simulink model "ECGdenoising_systemgenerator"  (R2018a)
settings: Solver=VariableStepAuto  StartTime=0.0  StopTime=10800  RelTol=1e-3
libraries: xbsIndex_r4 x811, dspsrcs4 x1
(part 1 of 3)
settings Model: Creator=NIKHIL  LastModifiedBy=NIKHIL

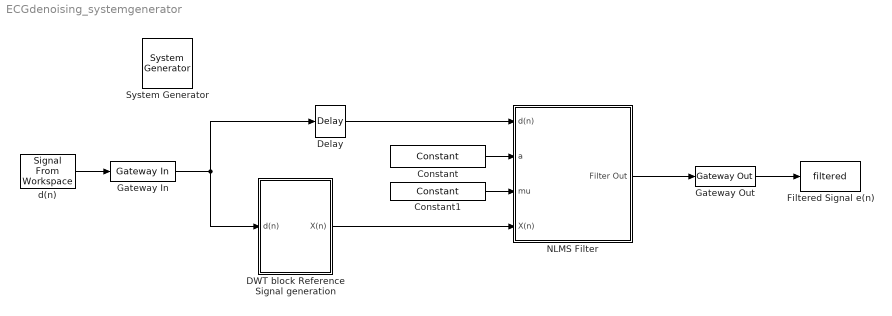
== system ECGdenoising_systemgenerator ==
  " System Generator" : xbsIndex_r4/ System Generator  Tag=genX  xilinxfamily=virtex7  part=xc7vx485t  speed=-2  package=ffg1761  synthesis_tool=Vivado  clock_wrapper=Clock Enables  directory=C:/Users/NIKHIL/Desktop/HDLCODE  proj_type=Vivado  Synth_file=Vivado Synthesis Defaults  Impl_file=Vivado Implementation Defaults  testbench=on  simulink_period=1  sysclk_period=10  dcm_input_clock_period=10  incr_netlist=off  trim_vbits=Everywhere in SubSystem  dbl_ovrd=According to Block Masks  core_generation=According to Block Masks  run_coregen=off  deprecated_control=off  eval_field=0  block_type=sysgen
  Constant : xbsIndex_r4/Constant  const=0.091  gui_display_data_type=Fixed-point  arith_type=Signed (2's comp)  n_bits=16  bin_pt=14  preci_type=Single  exp_width=8  frac_width=24  explicit_period=on  period=1  equ=P=C  opselect=C  inp2=PCIN>>17  opr=+  inp1=P  carry=CIN  dbl_ovrd=off  block_type=constant
  Constant1 : xbsIndex_r4/Constant  const=0.01  gui_display_data_type=Fixed-point  arith_type=Signed (2's comp)  n_bits=16  bin_pt=14  preci_type=Single  exp_width=8  frac_width=24  explicit_period=on  period=1  equ=P=C  opselect=C  inp2=PCIN>>17  opr=+  inp1=P  carry=CIN  dbl_ovrd=off  block_type=constant
  DWT block Reference Signal generation : Subsystem
  Delay : xbsIndex_r4/Delay  rst=off  infoeditControl=Selection of Reset will increase slice count due to use of real FFs and instead of SRLs  en=off  latency=889  reg_retiming=off  dbl_ovrd=off  block_type=delay
  Filtered Signal e(n) : ToWorkspace  VariableName=filtered  SampleTime=1
      settings: Save2DSignal=2-D array (concatenate along first dimension)
  Gateway In : xbsIndex_r4/Gateway In  gui_display_data_type=Fixed-point  arith_type="Signed  (2's comp)"  n_bits=16  bin_pt=14  preci_type=Single  exp_width=8  frac_width=24  rows=1  columns=1  quantization="Round  (unbiased: +/- Inf)"  overflow=Saturate  period=1  UseAsADC=off  ADCChannel='1'  interface=None  automatic_assignment=on  address_offset=hex2dec('00')  intf_name=''  intf_description=''  default_value=0  timing_constraint=None  locs_specified=off  LOCs={}  io_standard={}  inherit_from_input=off  hdl_port=on  dbl_ovrd=off  block_type=gatewayin
  Gateway Out : xbsIndex_r4/Gateway Out  inherit_from_input=off  hdl_port=on  rows=1  columns=1  UseAsDAC=off  DACChannel='1'  interface=None  automatic_assignment=on  address_offset=hex2dec('00')  intf_name=''  intf_description=''  timing_constraint=None  locs_specified=off  LOCs={}  io_standard={}  block_type=gatewayout
  NLMS Filter : Subsystem
  "d(n) " : dspsrcs4/Signal From Workspace  X=din  Ts=1  nsamps=1  OutputAfterFinalValue=Setting to zero  ignoreOrWarnInputAndFrameLengths=off  OutputFrames=off
  wires:
  Constant1/1 -> NLMS Filter/3(mu)
  NLMS Filter/1(Filter Out) -> Gateway Out/1
  "d(n) "/1 -> Gateway In/1
  Constant/1 -> NLMS Filter/2(a)
  DWT block Reference Signal generation/1(X(n)) -> NLMS Filter/4(X(n))
  Gateway Out/1 -> Filtered Signal e(n)/1
  Gateway In/1 -> DWT block Reference Signal generation/1("d(n) "), Delay/1
  Delay/1 -> NLMS Filter/1(d(n))

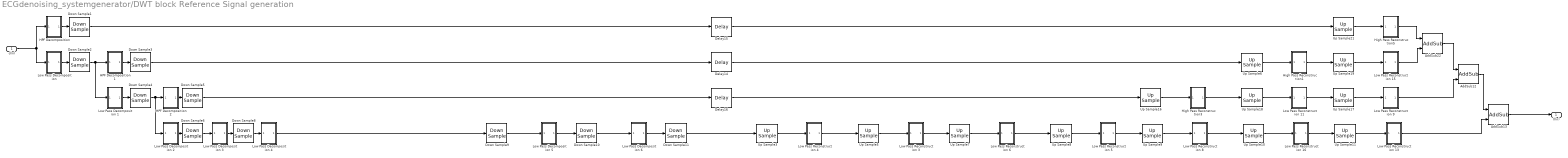
== system ECGdenoising_systemgenerator/DWT block Reference Signal generation ==
  "d(n) " : Inport  SampleTime=1
  AddSub12 : xbsIndex_r4/AddSub  mode=Addition  use_carryin=off  use_carryout=off  en=off  latency=0  precision=User Defined  arith_type="Signed  (2's comp)"  n_bits=16  bin_pt=14  quantization=Truncate  overflow=Saturate  use_behavioral_HDL=off  hw_selection=Fabric  pipelined=off  dbl_ovrd=off  block_type=addsub
  AddSub13 : xbsIndex_r4/AddSub  mode=Addition  use_carryin=off  use_carryout=off  en=off  latency=0  precision=User Defined  arith_type="Signed  (2's comp)"  n_bits=16  bin_pt=14  quantization=Truncate  overflow=Saturate  use_behavioral_HDL=off  hw_selection=Fabric  pipelined=off  dbl_ovrd=off  block_type=addsub
  AddSub22 : xbsIndex_r4/AddSub  mode=Addition  use_carryin=off  use_carryout=off  en=off  latency=0  precision=User Defined  arith_type="Signed  (2's comp)"  n_bits=16  bin_pt=14  quantization=Truncate  overflow=Saturate  use_behavioral_HDL=off  hw_selection=Fabric  pipelined=off  dbl_ovrd=off  block_type=addsub
  Delay14 : xbsIndex_r4/Delay  rst=off  infoeditControl=Selection of Reset will increase slice count due to use of real FFs and instead of SRLs  en=off  latency=217  reg_retiming=off  dbl_ovrd=off  block_type=delay
  Delay15 : xbsIndex_r4/Delay  rst=off  infoeditControl=Selection of Reset will increase slice count due to use of real FFs and instead of SRLs  en=off  latency=441  reg_retiming=off  dbl_ovrd=off  block_type=delay
  Delay16 : xbsIndex_r4/Delay  rst=off  infoeditControl=Selection of Reset will increase slice count due to use of real FFs and instead of SRLs  en=off  latency=105  reg_retiming=off  dbl_ovrd=off  block_type=delay
  Down Sample{1..6,8..11} (10 alike) : xbsIndex_r4/Down Sample  sample_ratio=2  sample_phase=First Value of Frame  en=off  rst=off  latency=0  dbl_ovrd=off  block_type=dsamp
  "HPF Decomposition " : Subsystem
  HPF Decomposition 1 : Subsystem
  HPF Decomposition 2 : Subsystem
  High Pass Reconstruction1 : Subsystem
  High Pass Reconstruction3 : Subsystem
  High Pass Reconstruction5 : Subsystem
  "Low Pass Decomposition " : Subsystem
  Low Pass Decomposition 1 : Subsystem
  Low Pass Decomposition 2 : Subsystem
  Low Pass Decomposition 3 : Subsystem
  Low Pass Decomposition 4 : Subsystem
  Low Pass Decomposition 5 : Subsystem
  Low Pass Decomposition 6 : Subsystem
  Low Pass Reconstruction 11 : Subsystem
  Low Pass Reconstruction 13 : Subsystem
  Low Pass Reconstruction 15 : Subsystem
  Low Pass Reconstruction 16 : Subsystem
  Low Pass Reconstruction 3 : Subsystem
  Low Pass Reconstruction 4 : Subsystem
  Low Pass Reconstruction 5 : Subsystem
  Low Pass Reconstruction 6 : Subsystem
  Low Pass Reconstruction 8 : Subsystem
  Low Pass Reconstruction 9 : Subsystem
  Up Sample{3,5..11,16..19,21} (13 alike) : xbsIndex_r4/Up Sample  sample_ratio=2  copy_samples=off  en=off  latency=0  dbl_ovrd=off  block_type=usamp
  X(n) : Outport  SampleTime=1
  wires:
  Down Sample3/1 -> Delay14/1
  Up Sample10/1 -> Low Pass Reconstruction 16/1(In3)
  AddSub22/1 -> AddSub12/1
  Down Sample5/1 -> Delay16/1
  Low Pass Reconstruction 15/1(Out3) -> AddSub22/2
  Up Sample6/1 -> High Pass Reconstruction1/1(In4)
  Low Pass Reconstruction 13/1(Out3) -> AddSub13/2
  Low Pass Reconstruction 5/1(Out3) -> Up Sample9/1
  Low Pass Reconstruction 9/1(Out3) -> AddSub12/2
  Up Sample11/1 -> Low Pass Reconstruction 13/1(In3)
  High Pass Reconstruction5/1(Out4) -> AddSub22/1
  Low Pass Reconstruction 8/1(Out3) -> Up Sample10/1
  High Pass Reconstruction1/1(Out4) -> Up Sample19/1
  AddSub13/1 -> X(n)/1
  Low Pass Reconstruction 3/1(Out3) -> Up Sample7/1
  Up Sample16/1 -> High Pass Reconstruction3/1(In4)
  Down Sample11/1 -> Up Sample3/1
  Up Sample8/1 -> Low Pass Reconstruction 5/1(In3)
  Up Sample18/1 -> Low Pass Reconstruction 11/1(In3)
  Delay15/1 -> Up Sample21/1
  Up Sample7/1 -> Low Pass Reconstruction 6/1(In3)
  Low Pass Reconstruction 6/1(Out3) -> Up Sample8/1
  Up Sample5/1 -> Low Pass Reconstruction 3/1(In3)
  Up Sample19/1 -> Low Pass Reconstruction 15/1(In3)
  Down Sample4/1 -> Low Pass Decomposition 2/1(In1), HPF Decomposition 2/1(In2)
  High Pass Reconstruction3/1(Out4) -> Up Sample18/1
  Up Sample3/1 -> Low Pass Reconstruction 4/1(In3)
  "HPF Decomposition "/1(Out2) -> Down Sample1/1
  Down Sample9/1 -> Low Pass Decomposition 5/1(In1)
  Low Pass Decomposition 4/1(Out1) -> Down Sample9/1
  Low Pass Reconstruction 16/1(Out3) -> Up Sample11/1
  Low Pass Decomposition 1/1(Out1) -> Down Sample4/1
  Down Sample8/1 -> Low Pass Decomposition 4/1(In1)
  Low Pass Decomposition 2/1(Out1) -> Down Sample6/1
  Low Pass Decomposition 3/1(Out1) -> Down Sample8/1
  Low Pass Decomposition 6/1(Out1) -> Down Sample11/1
  Up Sample21/1 -> High Pass Reconstruction5/1(In4)
  Low Pass Reconstruction 11/1(Out3) -> Up Sample17/1
  Low Pass Decomposition 5/1(Out1) -> Down Sample10/1
  Up Sample9/1 -> Low Pass Reconstruction 8/1(In3)
  Delay16/1 -> Up Sample16/1
  Down Sample2/1 -> Low Pass Decomposition 1/1(In1), HPF Decomposition 1/1(In2)
  HPF Decomposition 2/1(Out2) -> Down Sample5/1
  Delay14/1 -> Up Sample6/1
  AddSub12/1 -> AddSub13/1
  Up Sample17/1 -> Low Pass Reconstruction 9/1(In3)
  Down Sample10/1 -> Low Pass Decomposition 6/1(In1)
  Low Pass Reconstruction 4/1(Out3) -> Up Sample5/1
  "Low Pass Decomposition "/1(Out1) -> Down Sample2/1
  Down Sample1/1 -> Delay15/1
  "d(n) "/1 -> "HPF Decomposition "/1(In2), "Low Pass Decomposition "/1(In1)
  Down Sample6/1 -> Low Pass Decomposition 3/1(In1)
  HPF Decomposition 1/1(Out2) -> Down Sample3/1

== system ECGdenoising_systemgenerator/NLMS Filter ==
  note: e(n)
  d(n) : Inport  SampleTime=1
  a : Inport  Port=2  SampleTime=1
  mu : Inport  Port=3  SampleTime=1
  X(n) : Inport  Port=4  SampleTime=1
  12 tap FIR Filter : Subsystem
  AddSub12 : xbsIndex_r4/AddSub  mode=Subtraction  use_carryin=off  use_carryout=off  en=off  latency=0  precision=User Defined  arith_type="Signed  (2's comp)"  n_bits=16  bin_pt=14  quantization=Truncate  overflow=Saturate  use_behavioral_HDL=off  hw_selection=Fabric  pipelined=off  dbl_ovrd=off  block_type=addsub
  NLMS Algorithm : Subsystem
  Filter Out : Outport  SampleTime=1
  wires:
  NLMS Algorithm/4(coef4) -> 12 tap FIR Filter/5(Coeff4)
  NLMS Algorithm/9(coef9) -> 12 tap FIR Filter/10(Coeff9)
  mu/1 -> NLMS Algorithm/3(mu)
  AddSub12/1 -> Filter Out/1, NLMS Algorithm/1(e(n))
  12 tap FIR Filter/1(Y(n)) -> AddSub12/2
  X(n)/1 -> 12 tap FIR Filter/1("X(n) "), NLMS Algorithm/4(X(n))
  NLMS Algorithm/10(coef10) -> 12 tap FIR Filter/11(Coeff10)
  NLMS Algorithm/2(coef2) -> 12 tap FIR Filter/3(Coeff2)
  NLMS Algorithm/8(coef8) -> 12 tap FIR Filter/9(Coeff8)
  NLMS Algorithm/6(coef6) -> 12 tap FIR Filter/7(Coeff6)
  NLMS Algorithm/11(coef11) -> 12 tap FIR Filter/12(Coeff11)
  NLMS Algorithm/5(coef5) -> 12 tap FIR Filter/6(Coeff5)
  NLMS Algorithm/7(coef7) -> 12 tap FIR Filter/8(Coeff7)
  NLMS Algorithm/1(coef1) -> 12 tap FIR Filter/2(Coeff1)
  d(n)/1 -> AddSub12/1
  NLMS Algorithm/12(coef12) -> 12 tap FIR Filter/13(Coeff12)
  NLMS Algorithm/3(coef3) -> 12 tap FIR Filter/4(Coeff3)
  a/1 -> NLMS Algorithm/2(a)

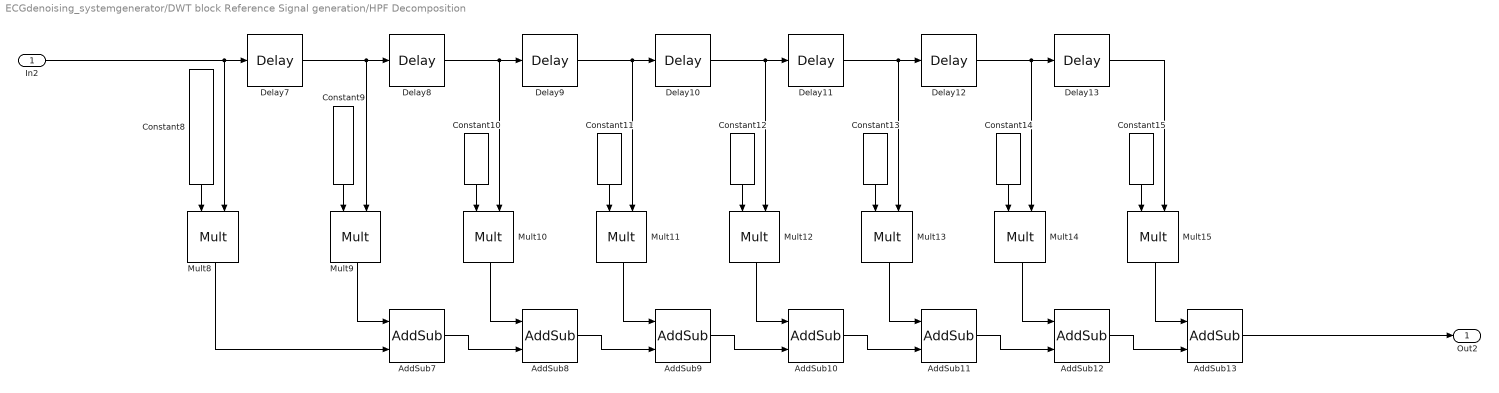
== system ECGdenoising_systemgenerator/DWT block Reference Signal generation/HPF Decomposition  ==
  In2 : Inport
  AddSub{7..13} (7 alike) : xbsIndex_r4/AddSub  mode=Addition  use_carryin=off  use_carryout=off  en=off  latency=0  precision=User Defined  arith_type="Signed  (2's comp)"  n_bits=16  bin_pt=14  quantization=Truncate  overflow=Saturate  use_behavioral_HDL=off  hw_selection=Fabric  pipelined=off  dbl_ovrd=off  block_type=addsub
  Constant10 : xbsIndex_r4/Constant  const=-0.6308807679  gui_display_data_type=Fixed-point  arith_type=Signed (2's comp)  n_bits=16  bin_pt=14  preci_type=Single  exp_width=8  frac_width=24  explicit_period=on  period=1  equ=P=C  opselect=C  inp2=PCIN>>17  opr=+  inp1=P  carry=CIN  dbl_ovrd=off  block_type=constant
  Constant11 : xbsIndex_r4/Constant  const=-0.0279837694  gui_display_data_type=Fixed-point  arith_type=Signed (2's comp)  n_bits=16  bin_pt=14  preci_type=Single  exp_width=8  frac_width=24  explicit_period=on  period=1  equ=P=C  opselect=C  inp2=PCIN>>17  opr=+  inp1=P  carry=CIN  dbl_ovrd=off  block_type=constant
  Constant12 : xbsIndex_r4/Constant  const=0.1870348117  gui_display_data_type=Fixed-point  arith_type=Signed (2's comp)  n_bits=16  bin_pt=14  preci_type=Single  exp_width=8  frac_width=24  explicit_period=on  period=1  equ=P=C  opselect=C  inp2=PCIN>>17  opr=+  inp1=P  carry=CIN  dbl_ovrd=off  block_type=constant
  Constant13 : xbsIndex_r4/Constant  const=0.0308413818  gui_display_data_type=Fixed-point  arith_type=Signed (2's comp)  n_bits=16  bin_pt=14  preci_type=Single  exp_width=8  frac_width=24  explicit_period=on  period=1  equ=P=C  opselect=C  inp2=PCIN>>17  opr=+  inp1=P  carry=CIN  dbl_ovrd=off  block_type=constant
  Constant14 : xbsIndex_r4/Constant  const=-0.0328830117  gui_display_data_type=Fixed-point  arith_type=Signed (2's comp)  n_bits=16  bin_pt=14  preci_type=Single  exp_width=8  frac_width=24  explicit_period=on  period=1  equ=P=C  opselect=C  inp2=PCIN>>17  opr=+  inp1=P  carry=CIN  dbl_ovrd=off  block_type=constant
  Constant15 : xbsIndex_r4/Constant  const=-0.0105974018  gui_display_data_type=Fixed-point  arith_type=Signed (2's comp)  n_bits=16  bin_pt=14  preci_type=Single  exp_width=8  frac_width=24  explicit_period=on  period=1  equ=P=C  opselect=C  inp2=PCIN>>17  opr=+  inp1=P  carry=CIN  dbl_ovrd=off  block_type=constant
  Constant8 : xbsIndex_r4/Constant  const=-0.2303778133  gui_display_data_type=Fixed-point  arith_type=Signed (2's comp)  n_bits=16  bin_pt=14  preci_type=Single  exp_width=8  frac_width=24  explicit_period=on  period=1  equ=P=C  opselect=C  inp2=PCIN>>17  opr=+  inp1=P  carry=CIN  dbl_ovrd=off  block_type=constant
  Constant9 : xbsIndex_r4/Constant  const=0.7148465706  gui_display_data_type=Fixed-point  arith_type=Signed (2's comp)  n_bits=16  bin_pt=14  preci_type=Single  exp_width=8  frac_width=24  explicit_period=on  period=1  equ=P=C  opselect=C  inp2=PCIN>>17  opr=+  inp1=P  carry=CIN  dbl_ovrd=off  block_type=constant
  Delay{7..13} (7 alike) : xbsIndex_r4/Delay  rst=off  infoeditControl=Selection of Reset will increase slice count due to use of real FFs and instead of SRLs  en=off  latency=1  reg_retiming=off  dbl_ovrd=off  block_type=delay
      Delay10 settings: infoedit=Hardware notes: A delay line is a chain, each link of which is an SRL16 or SRL32 followed by a flip-flop.
      Delay11 settings: infoedit=Hardware notes: A delay line is a chain, each link of which is an SRL16 or SRL32 followed by a flip-flop.
      Delay12 settings: infoedit=Hardware notes: A delay line is a chain, each link of which is an SRL16 or SRL32 followed by a flip-flop.
      Delay13 settings: infoedit=Hardware notes: A delay line is a chain, each link of which is an SRL16 or SRL32 followed by a flip-flop.
      Delay7 settings: infoedit=Hardware notes: A delay line is a chain, each link of which is an SRL16 or SRL32 followed by a flip-flop.
      Delay8 settings: infoedit=Hardware notes: A delay line is a chain, each link of which is an SRL16 or SRL32 followed by a flip-flop.
  Mult{8..15} (8 alike) : xbsIndex_r4/Mult  precision=User Defined  arith_type="Signed  (2's comp)"  n_bits=32  bin_pt=28  quantization=Truncate  overflow=Saturate  en=off  latency=0  use_behavioral_HDL=off  opt=Speed  use_embedded=on  optimum_pipeline=off  pipeline=on  dbl_ovrd=off  use_rpm=on  placement_style=Triangular  block_type=mult
  Out2 : Outport
  wires:
  Constant8/1 -> Mult8/1
  Constant9/1 -> Mult9/1
  Constant10/1 -> Mult10/1
  Mult10/1 -> AddSub8/1
  AddSub7/1 -> AddSub8/2
  Delay9/1 -> Mult11/2, Delay10/1
  Constant11/1 -> Mult11/1
  Mult11/1 -> AddSub9/1
  AddSub8/1 -> AddSub9/2
  Mult8/1 -> AddSub7/2
  Delay10/1 -> Mult12/2, Delay11/1
  Delay7/1 -> Mult9/2, Delay8/1
  Mult9/1 -> AddSub7/1
  In2/1 -> Mult8/2, Delay7/1
  Delay8/1 -> Mult10/2, Delay9/1
  Constant13/1 -> Mult13/1
  Delay13/1 -> Mult15/2
  Constant15/1 -> Mult15/1
  Mult15/1 -> AddSub13/1
  Mult13/1 -> AddSub11/1
  AddSub9/1 -> AddSub10/2
  Mult14/1 -> AddSub12/1
  AddSub11/1 -> AddSub12/2
  Mult12/1 -> AddSub10/1
  Delay11/1 -> Mult13/2, Delay12/1
  AddSub10/1 -> AddSub11/2
  Constant14/1 -> Mult14/1
  AddSub12/1 -> AddSub13/2
  Constant12/1 -> Mult12/1
  Delay12/1 -> Mult14/2, Delay13/1
  AddSub13/1 -> Out2/1

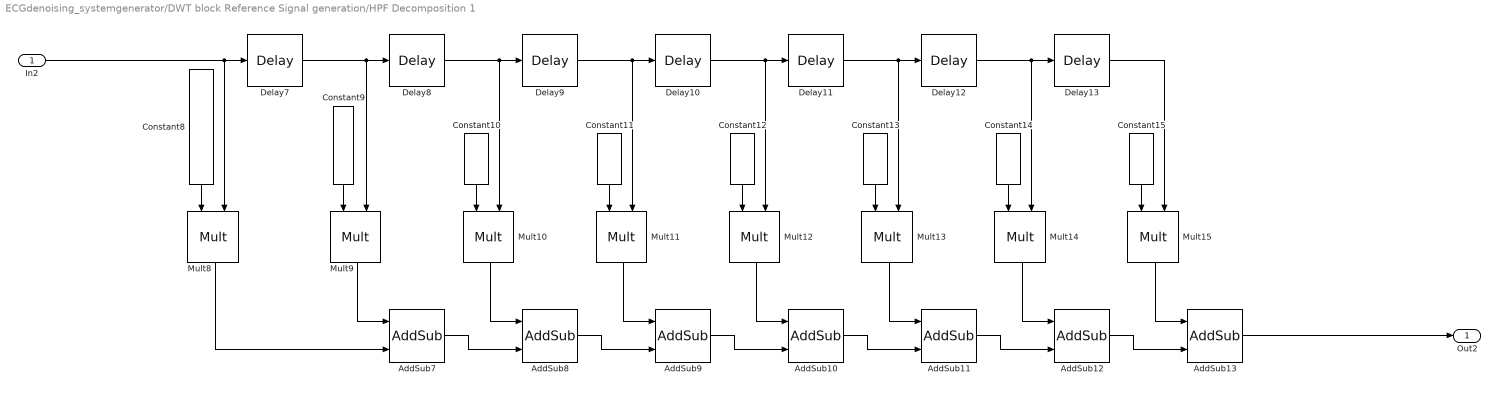
== system ECGdenoising_systemgenerator/DWT block Reference Signal generation/HPF Decomposition 1 ==
  In2 : Inport
  AddSub{7..13} (7 alike) : xbsIndex_r4/AddSub  mode=Addition  use_carryin=off  use_carryout=off  en=off  latency=0  precision=User Defined  arith_type="Signed  (2's comp)"  n_bits=16  bin_pt=14  quantization=Truncate  overflow=Saturate  use_behavioral_HDL=off  hw_selection=Fabric  pipelined=off  dbl_ovrd=off  block_type=addsub
  Constant10 : xbsIndex_r4/Constant  const=-0.6308807679  gui_display_data_type=Fixed-point  arith_type=Signed (2's comp)  n_bits=16  bin_pt=14  preci_type=Single  exp_width=8  frac_width=24  explicit_period=on  period=2  equ=P=C  opselect=C  inp2=PCIN>>17  opr=+  inp1=P  carry=CIN  dbl_ovrd=off  block_type=constant
  Constant11 : xbsIndex_r4/Constant  const=-0.0279837694  gui_display_data_type=Fixed-point  arith_type=Signed (2's comp)  n_bits=16  bin_pt=14  preci_type=Single  exp_width=8  frac_width=24  explicit_period=on  period=2  equ=P=C  opselect=C  inp2=PCIN>>17  opr=+  inp1=P  carry=CIN  dbl_ovrd=off  block_type=constant
  Constant12 : xbsIndex_r4/Constant  const=0.1870348117  gui_display_data_type=Fixed-point  arith_type=Signed (2's comp)  n_bits=16  bin_pt=14  preci_type=Single  exp_width=8  frac_width=24  explicit_period=on  period=2  equ=P=C  opselect=C  inp2=PCIN>>17  opr=+  inp1=P  carry=CIN  dbl_ovrd=off  block_type=constant
  Constant13 : xbsIndex_r4/Constant  const=0.0308413818  gui_display_data_type=Fixed-point  arith_type=Signed (2's comp)  n_bits=16  bin_pt=14  preci_type=Single  exp_width=8  frac_width=24  explicit_period=on  period=2  equ=P=C  opselect=C  inp2=PCIN>>17  opr=+  inp1=P  carry=CIN  dbl_ovrd=off  block_type=constant
  Constant14 : xbsIndex_r4/Constant  const=-0.0328830117  gui_display_data_type=Fixed-point  arith_type=Signed (2's comp)  n_bits=16  bin_pt=14  preci_type=Single  exp_width=8  frac_width=24  explicit_period=on  period=2  equ=P=C  opselect=C  inp2=PCIN>>17  opr=+  inp1=P  carry=CIN  dbl_ovrd=off  block_type=constant
  Constant15 : xbsIndex_r4/Constant  const=-0.0105974018  gui_display_data_type=Fixed-point  arith_type=Signed (2's comp)  n_bits=16  bin_pt=14  preci_type=Single  exp_width=8  frac_width=24  explicit_period=on  period=2  equ=P=C  opselect=C  inp2=PCIN>>17  opr=+  inp1=P  carry=CIN  dbl_ovrd=off  block_type=constant
  Constant8 : xbsIndex_r4/Constant  const=-0.2303778133  gui_display_data_type=Fixed-point  arith_type=Signed (2's comp)  n_bits=16  bin_pt=14  preci_type=Single  exp_width=8  frac_width=24  explicit_period=on  period=2  equ=P=C  opselect=C  inp2=PCIN>>17  opr=+  inp1=P  carry=CIN  dbl_ovrd=off  block_type=constant
  Constant9 : xbsIndex_r4/Constant  const=0.7148465706  gui_display_data_type=Fixed-point  arith_type=Signed (2's comp)  n_bits=16  bin_pt=14  preci_type=Single  exp_width=8  frac_width=24  explicit_period=on  period=2  equ=P=C  opselect=C  inp2=PCIN>>17  opr=+  inp1=P  carry=CIN  dbl_ovrd=off  block_type=constant
  Delay{7..13} (7 alike) : xbsIndex_r4/Delay  rst=off  infoeditControl=Selection of Reset will increase slice count due to use of real FFs and instead of SRLs  en=off  latency=1  reg_retiming=off  dbl_ovrd=off  block_type=delay
      settings: infoedit=Hardware notes: A delay line is a chain, each link of which is an SRL16 or SRL32 followed by a flip-flop.
  Mult{8..15} (8 alike) : xbsIndex_r4/Mult  precision=User Defined  arith_type="Signed  (2's comp)"  n_bits=32  bin_pt=28  quantization=Truncate  overflow=Saturate  en=off  latency=0  use_behavioral_HDL=off  opt=Speed  use_embedded=on  optimum_pipeline=off  pipeline=on  dbl_ovrd=off  use_rpm=on  placement_style=Triangular  block_type=mult
  Out2 : Outport
  wires:
  Constant8/1 -> Mult8/1
  Constant9/1 -> Mult9/1
  Constant10/1 -> Mult10/1
  Mult10/1 -> AddSub8/1
  AddSub7/1 -> AddSub8/2
  Delay9/1 -> Mult11/2, Delay10/1
  Constant11/1 -> Mult11/1
  Mult11/1 -> AddSub9/1
  AddSub8/1 -> AddSub9/2
  Mult8/1 -> AddSub7/2
  Delay10/1 -> Mult12/2, Delay11/1
  Delay7/1 -> Mult9/2, Delay8/1
  Mult9/1 -> AddSub7/1
  In2/1 -> Mult8/2, Delay7/1
  Delay8/1 -> Mult10/2, Delay9/1
  Constant13/1 -> Mult13/1
  Delay13/1 -> Mult15/2
  Constant15/1 -> Mult15/1
  Mult15/1 -> AddSub13/1
  Mult13/1 -> AddSub11/1
  AddSub9/1 -> AddSub10/2
  Mult14/1 -> AddSub12/1
  AddSub11/1 -> AddSub12/2
  Mult12/1 -> AddSub10/1
  Delay11/1 -> Mult13/2, Delay12/1
  AddSub10/1 -> AddSub11/2
  Constant14/1 -> Mult14/1
  AddSub12/1 -> AddSub13/2
  Constant12/1 -> Mult12/1
  Delay12/1 -> Mult14/2, Delay13/1
  AddSub13/1 -> Out2/1

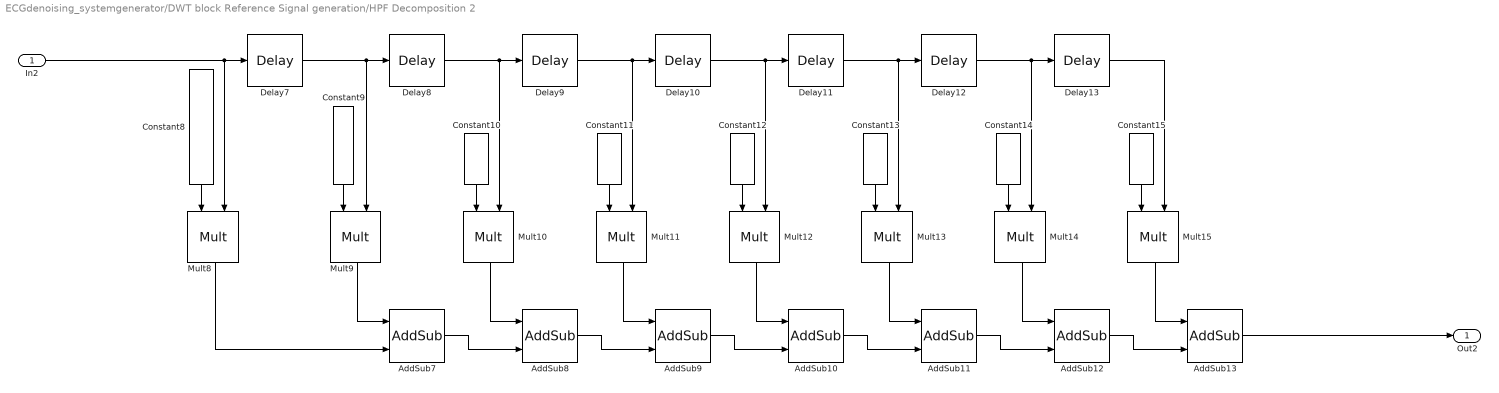
== system ECGdenoising_systemgenerator/DWT block Reference Signal generation/HPF Decomposition 2 ==
  In2 : Inport
  AddSub{7..13} (7 alike) : xbsIndex_r4/AddSub  mode=Addition  use_carryin=off  use_carryout=off  en=off  latency=0  precision=User Defined  arith_type="Signed  (2's comp)"  n_bits=16  bin_pt=14  quantization=Truncate  overflow=Saturate  use_behavioral_HDL=off  hw_selection=Fabric  pipelined=off  dbl_ovrd=off  block_type=addsub
  Constant10 : xbsIndex_r4/Constant  const=-0.6308807679  gui_display_data_type=Fixed-point  arith_type=Signed (2's comp)  n_bits=16  bin_pt=14  preci_type=Single  exp_width=8  frac_width=24  explicit_period=on  period=4  equ=P=C  opselect=C  inp2=PCIN>>17  opr=+  inp1=P  carry=CIN  dbl_ovrd=off  block_type=constant
  Constant11 : xbsIndex_r4/Constant  const=-0.0279837694  gui_display_data_type=Fixed-point  arith_type=Signed (2's comp)  n_bits=16  bin_pt=14  preci_type=Single  exp_width=8  frac_width=24  explicit_period=on  period=4  equ=P=C  opselect=C  inp2=PCIN>>17  opr=+  inp1=P  carry=CIN  dbl_ovrd=off  block_type=constant
  Constant12 : xbsIndex_r4/Constant  const=0.1870348117  gui_display_data_type=Fixed-point  arith_type=Signed (2's comp)  n_bits=16  bin_pt=14  preci_type=Single  exp_width=8  frac_width=24  explicit_period=on  period=4  equ=P=C  opselect=C  inp2=PCIN>>17  opr=+  inp1=P  carry=CIN  dbl_ovrd=off  block_type=constant
  Constant13 : xbsIndex_r4/Constant  const=0.0308413818  gui_display_data_type=Fixed-point  arith_type=Signed (2's comp)  n_bits=16  bin_pt=14  preci_type=Single  exp_width=8  frac_width=24  explicit_period=on  period=4  equ=P=C  opselect=C  inp2=PCIN>>17  opr=+  inp1=P  carry=CIN  dbl_ovrd=off  block_type=constant
  Constant14 : xbsIndex_r4/Constant  const=-0.0328830117  gui_display_data_type=Fixed-point  arith_type=Signed (2's comp)  n_bits=16  bin_pt=14  preci_type=Single  exp_width=8  frac_width=24  explicit_period=on  period=4  equ=P=C  opselect=C  inp2=PCIN>>17  opr=+  inp1=P  carry=CIN  dbl_ovrd=off  block_type=constant
  Constant15 : xbsIndex_r4/Constant  const=-0.0105974018  gui_display_data_type=Fixed-point  arith_type=Signed (2's comp)  n_bits=16  bin_pt=14  preci_type=Single  exp_width=8  frac_width=24  explicit_period=on  period=4  equ=P=C  opselect=C  inp2=PCIN>>17  opr=+  inp1=P  carry=CIN  dbl_ovrd=off  block_type=constant
  Constant8 : xbsIndex_r4/Constant  const=-0.2303778133  gui_display_data_type=Fixed-point  arith_type=Signed (2's comp)  n_bits=16  bin_pt=14  preci_type=Single  exp_width=8  frac_width=24  explicit_period=on  period=4  equ=P=C  opselect=C  inp2=PCIN>>17  opr=+  inp1=P  carry=CIN  dbl_ovrd=off  block_type=constant
  Constant9 : xbsIndex_r4/Constant  const=0.7148465706  gui_display_data_type=Fixed-point  arith_type=Signed (2's comp)  n_bits=16  bin_pt=14  preci_type=Single  exp_width=8  frac_width=24  explicit_period=on  period=4  equ=P=C  opselect=C  inp2=PCIN>>17  opr=+  inp1=P  carry=CIN  dbl_ovrd=off  block_type=constant
  Delay{7..13} (7 alike) : xbsIndex_r4/Delay  rst=off  infoeditControl=Selection of Reset will increase slice count due to use of real FFs and instead of SRLs  en=off  latency=1  reg_retiming=off  dbl_ovrd=off  block_type=delay
      settings: infoedit=Hardware notes: A delay line is a chain, each link of which is an SRL16 or SRL32 followed by a flip-flop.
  Mult{8..15} (8 alike) : xbsIndex_r4/Mult  precision=User Defined  arith_type="Signed  (2's comp)"  n_bits=32  bin_pt=28  quantization=Truncate  overflow=Saturate  en=off  latency=0  use_behavioral_HDL=off  opt=Speed  use_embedded=on  optimum_pipeline=off  pipeline=on  dbl_ovrd=off  use_rpm=on  placement_style=Triangular  block_type=mult
  Out2 : Outport
  wires:
  Constant8/1 -> Mult8/1
  Constant9/1 -> Mult9/1
  Constant10/1 -> Mult10/1
  Mult10/1 -> AddSub8/1
  AddSub7/1 -> AddSub8/2
  Delay9/1 -> Mult11/2, Delay10/1
  Constant11/1 -> Mult11/1
  Mult11/1 -> AddSub9/1
  AddSub8/1 -> AddSub9/2
  Mult8/1 -> AddSub7/2
  Delay10/1 -> Mult12/2, Delay11/1
  Delay7/1 -> Mult9/2, Delay8/1
  Mult9/1 -> AddSub7/1
  In2/1 -> Mult8/2, Delay7/1
  Delay8/1 -> Mult10/2, Delay9/1
  Constant13/1 -> Mult13/1
  Delay13/1 -> Mult15/2
  Constant15/1 -> Mult15/1
  Mult15/1 -> AddSub13/1
  Mult13/1 -> AddSub11/1
  AddSub9/1 -> AddSub10/2
  Mult14/1 -> AddSub12/1
  AddSub11/1 -> AddSub12/2
  Mult12/1 -> AddSub10/1
  Delay11/1 -> Mult13/2, Delay12/1
  AddSub10/1 -> AddSub11/2
  Constant14/1 -> Mult14/1
  AddSub12/1 -> AddSub13/2
  Constant12/1 -> Mult12/1
  Delay12/1 -> Mult14/2, Delay13/1
  AddSub13/1 -> Out2/1

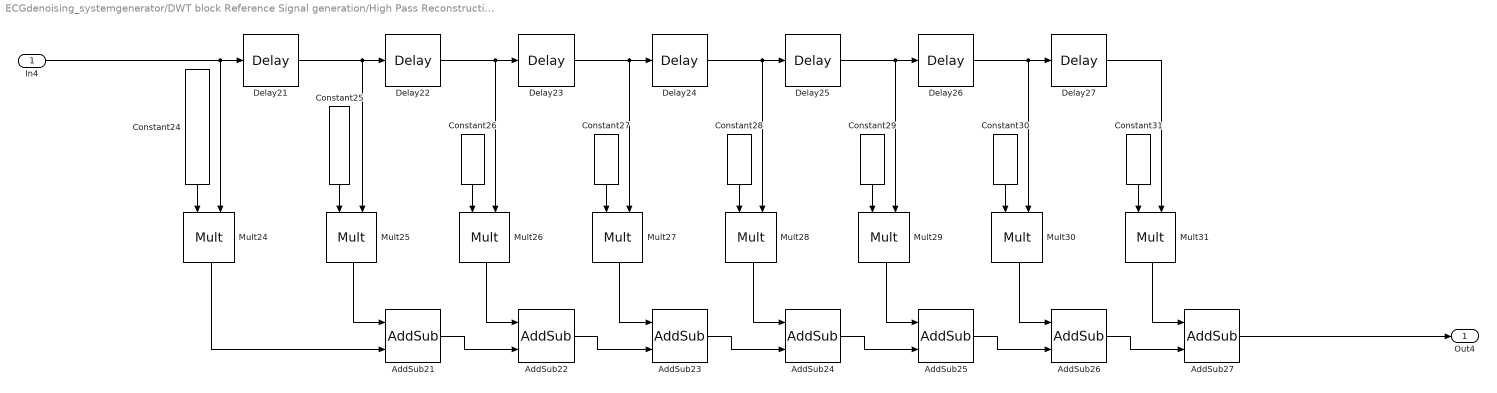
== system ECGdenoising_systemgenerator/DWT block Reference Signal generation/High Pass Reconstruction1 ==
  In4 : Inport
  AddSub{21..27} (7 alike) : xbsIndex_r4/AddSub  mode=Addition  use_carryin=off  use_carryout=off  en=off  latency=0  precision=User Defined  arith_type="Signed  (2's comp)"  n_bits=16  bin_pt=14  quantization=Truncate  overflow=Saturate  use_behavioral_HDL=off  hw_selection=Fabric  pipelined=off  dbl_ovrd=off  block_type=addsub
  Constant24 : xbsIndex_r4/Constant  const=-0.0105974018  gui_display_data_type=Fixed-point  arith_type=Signed (2's comp)  n_bits=16  bin_pt=14  preci_type=Single  exp_width=8  frac_width=24  explicit_period=on  period=2  equ=P=C  opselect=C  inp2=PCIN>>17  opr=+  inp1=P  carry=CIN  dbl_ovrd=off  block_type=constant
  Constant25 : xbsIndex_r4/Constant  const=-0.032883011  gui_display_data_type=Fixed-point  arith_type=Signed (2's comp)  n_bits=16  bin_pt=14  preci_type=Single  exp_width=8  frac_width=24  explicit_period=on  period=2  equ=P=C  opselect=C  inp2=PCIN>>17  opr=+  inp1=P  carry=CIN  dbl_ovrd=off  block_type=constant
  Constant26 : xbsIndex_r4/Constant  const=0.0308413818  gui_display_data_type=Fixed-point  arith_type=Signed (2's comp)  n_bits=16  bin_pt=14  preci_type=Single  exp_width=8  frac_width=24  explicit_period=on  period=2  equ=P=C  opselect=C  inp2=PCIN>>17  opr=+  inp1=P  carry=CIN  dbl_ovrd=off  block_type=constant
  Constant27 : xbsIndex_r4/Constant  const=0.1870348117  gui_display_data_type=Fixed-point  arith_type=Signed (2's comp)  n_bits=16  bin_pt=14  preci_type=Single  exp_width=8  frac_width=24  explicit_period=on  period=2  equ=P=C  opselect=C  inp2=PCIN>>17  opr=+  inp1=P  carry=CIN  dbl_ovrd=off  block_type=constant
  Constant28 : xbsIndex_r4/Constant  const=-0.0279837694  gui_display_data_type=Fixed-point  arith_type=Signed (2's comp)  n_bits=16  bin_pt=14  preci_type=Single  exp_width=8  frac_width=24  explicit_period=on  period=2  equ=P=C  opselect=C  inp2=PCIN>>17  opr=+  inp1=P  carry=CIN  dbl_ovrd=off  block_type=constant
  Constant29 : xbsIndex_r4/Constant  const=-0.6308807679  gui_display_data_type=Fixed-point  arith_type=Signed (2's comp)  n_bits=16  bin_pt=14  preci_type=Single  exp_width=8  frac_width=24  explicit_period=on  period=2  equ=P=C  opselect=C  inp2=PCIN>>17  opr=+  inp1=P  carry=CIN  dbl_ovrd=off  block_type=constant
  Constant30 : xbsIndex_r4/Constant  const=0.7148465706  gui_display_data_type=Fixed-point  arith_type=Signed (2's comp)  n_bits=16  bin_pt=14  preci_type=Single  exp_width=8  frac_width=24  explicit_period=on  period=2  equ=P=C  opselect=C  inp2=PCIN>>17  opr=+  inp1=P  carry=CIN  dbl_ovrd=off  block_type=constant
  Constant31 : xbsIndex_r4/Constant  const=-0.2303778133  gui_display_data_type=Fixed-point  arith_type=Signed (2's comp)  n_bits=16  bin_pt=14  preci_type=Single  exp_width=8  frac_width=24  explicit_period=on  period=2  equ=P=C  opselect=C  inp2=PCIN>>17  opr=+  inp1=P  carry=CIN  dbl_ovrd=off  block_type=constant
  Delay{21..27} (7 alike) : xbsIndex_r4/Delay  rst=off  infoeditControl=Selection of Reset will increase slice count due to use of real FFs and instead of SRLs  en=off  latency=1  reg_retiming=off  dbl_ovrd=off  block_type=delay
      settings: infoedit=Hardware notes: A delay line is a chain, each link of which is an SRL16 or SRL32 followed by a flip-flop.
  Mult{24..31} (8 alike) : xbsIndex_r4/Mult  precision=User Defined  arith_type="Signed  (2's comp)"  n_bits=32  bin_pt=28  quantization=Truncate  overflow=Saturate  en=off  latency=0  use_behavioral_HDL=off  opt=Speed  use_embedded=on  optimum_pipeline=off  pipeline=on  dbl_ovrd=off  use_rpm=on  placement_style=Triangular  block_type=mult
  Out4 : Outport
  wires:
  Delay21/1 -> Mult25/2, Delay22/1
  Delay22/1 -> Mult26/2, Delay23/1
  Delay23/1 -> Mult27/2, Delay24/1
  AddSub21/1 -> AddSub22/2
  AddSub23/1 -> AddSub24/2
  In4/1 -> Mult24/2, Delay21/1
  Mult29/1 -> AddSub25/1
  Constant25/1 -> Mult25/1
  Delay24/1 -> Mult28/2, Delay25/1
  Mult27/1 -> AddSub23/1
  Mult28/1 -> AddSub24/1
  AddSub24/1 -> AddSub25/2
  Mult26/1 -> AddSub22/1
  Delay26/1 -> Mult30/2, Delay27/1
  AddSub22/1 -> AddSub23/2
  Delay25/1 -> Mult29/2, Delay26/1
  Mult25/1 -> AddSub21/1
  Mult30/1 -> AddSub26/1
  AddSub25/1 -> AddSub26/2
  Constant29/1 -> Mult29/1
  Constant27/1 -> Mult27/1
  Mult24/1 -> AddSub21/2
  Constant28/1 -> Mult28/1
  Delay27/1 -> Mult31/2
  Constant31/1 -> Mult31/1
  Constant24/1 -> Mult24/1
  Constant30/1 -> Mult30/1
  Constant26/1 -> Mult26/1
  Mult31/1 -> AddSub27/1
  AddSub26/1 -> AddSub27/2
  AddSub27/1 -> Out4/1

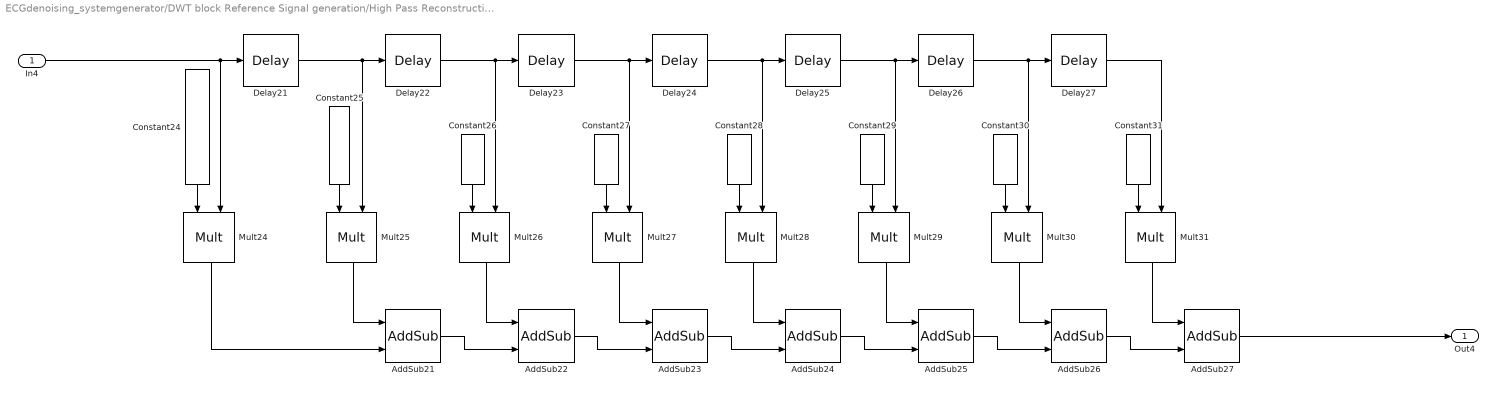
== system ECGdenoising_systemgenerator/DWT block Reference Signal generation/High Pass Reconstruction3 ==
  In4 : Inport
  AddSub{21..27} (7 alike) : xbsIndex_r4/AddSub  mode=Addition  use_carryin=off  use_carryout=off  en=off  latency=0  precision=User Defined  arith_type="Signed  (2's comp)"  n_bits=16  bin_pt=14  quantization=Truncate  overflow=Saturate  use_behavioral_HDL=off  hw_selection=Fabric  pipelined=off  dbl_ovrd=off  block_type=addsub
  Constant24 : xbsIndex_r4/Constant  const=-0.0105974018  gui_display_data_type=Fixed-point  arith_type=Signed (2's comp)  n_bits=16  bin_pt=14  preci_type=Single  exp_width=8  frac_width=24  explicit_period=on  period=4  equ=P=C  opselect=C  inp2=PCIN>>17  opr=+  inp1=P  carry=CIN  dbl_ovrd=off  block_type=constant
  Constant25 : xbsIndex_r4/Constant  const=-0.032883011  gui_display_data_type=Fixed-point  arith_type=Signed (2's comp)  n_bits=16  bin_pt=14  preci_type=Single  exp_width=8  frac_width=24  explicit_period=on  period=4  equ=P=C  opselect=C  inp2=PCIN>>17  opr=+  inp1=P  carry=CIN  dbl_ovrd=off  block_type=constant
  Constant26 : xbsIndex_r4/Constant  const=0.0308413818  gui_display_data_type=Fixed-point  arith_type=Signed (2's comp)  n_bits=16  bin_pt=14  preci_type=Single  exp_width=8  frac_width=24  explicit_period=on  period=4  equ=P=C  opselect=C  inp2=PCIN>>17  opr=+  inp1=P  carry=CIN  dbl_ovrd=off  block_type=constant
  Constant27 : xbsIndex_r4/Constant  const=0.1870348117  gui_display_data_type=Fixed-point  arith_type=Signed (2's comp)  n_bits=16  bin_pt=14  preci_type=Single  exp_width=8  frac_width=24  explicit_period=on  period=4  equ=P=C  opselect=C  inp2=PCIN>>17  opr=+  inp1=P  carry=CIN  dbl_ovrd=off  block_type=constant
  Constant28 : xbsIndex_r4/Constant  const=-0.0279837694  gui_display_data_type=Fixed-point  arith_type=Signed (2's comp)  n_bits=16  bin_pt=14  preci_type=Single  exp_width=8  frac_width=24  explicit_period=on  period=4  equ=P=C  opselect=C  inp2=PCIN>>17  opr=+  inp1=P  carry=CIN  dbl_ovrd=off  block_type=constant
  Constant29 : xbsIndex_r4/Constant  const=-0.6308807679  gui_display_data_type=Fixed-point  arith_type=Signed (2's comp)  n_bits=16  bin_pt=14  preci_type=Single  exp_width=8  frac_width=24  explicit_period=on  period=4  equ=P=C  opselect=C  inp2=PCIN>>17  opr=+  inp1=P  carry=CIN  dbl_ovrd=off  block_type=constant
  Constant30 : xbsIndex_r4/Constant  const=0.7148465706  gui_display_data_type=Fixed-point  arith_type=Signed (2's comp)  n_bits=16  bin_pt=14  preci_type=Single  exp_width=8  frac_width=24  explicit_period=on  period=4  equ=P=C  opselect=C  inp2=PCIN>>17  opr=+  inp1=P  carry=CIN  dbl_ovrd=off  block_type=constant
  Constant31 : xbsIndex_r4/Constant  const=-0.2303778133  gui_display_data_type=Fixed-point  arith_type=Signed (2's comp)  n_bits=16  bin_pt=14  preci_type=Single  exp_width=8  frac_width=24  explicit_period=on  period=4  equ=P=C  opselect=C  inp2=PCIN>>17  opr=+  inp1=P  carry=CIN  dbl_ovrd=off  block_type=constant
  Delay{21..27} (7 alike) : xbsIndex_r4/Delay  rst=off  infoeditControl=Selection of Reset will increase slice count due to use of real FFs and instead of SRLs  en=off  latency=1  reg_retiming=off  dbl_ovrd=off  block_type=delay
      settings: infoedit=Hardware notes: A delay line is a chain, each link of which is an SRL16 or SRL32 followed by a flip-flop.
  Mult{24..31} (8 alike) : xbsIndex_r4/Mult  precision=User Defined  arith_type="Signed  (2's comp)"  n_bits=32  bin_pt=28  quantization=Truncate  overflow=Saturate  en=off  latency=0  use_behavioral_HDL=off  opt=Speed  use_embedded=on  optimum_pipeline=off  pipeline=on  dbl_ovrd=off  use_rpm=on  placement_style=Triangular  block_type=mult
  Out4 : Outport
  wires:
  Delay21/1 -> Mult25/2, Delay22/1
  Delay22/1 -> Mult26/2, Delay23/1
  Delay23/1 -> Mult27/2, Delay24/1
  AddSub21/1 -> AddSub22/2
  AddSub23/1 -> AddSub24/2
  In4/1 -> Mult24/2, Delay21/1
  Mult29/1 -> AddSub25/1
  Constant25/1 -> Mult25/1
  Delay24/1 -> Mult28/2, Delay25/1
  Mult27/1 -> AddSub23/1
  Mult28/1 -> AddSub24/1
  AddSub24/1 -> AddSub25/2
  Mult26/1 -> AddSub22/1
  Delay26/1 -> Mult30/2, Delay27/1
  AddSub22/1 -> AddSub23/2
  Delay25/1 -> Mult29/2, Delay26/1
  Mult25/1 -> AddSub21/1
  Mult30/1 -> AddSub26/1
  AddSub25/1 -> AddSub26/2
  Constant29/1 -> Mult29/1
  Constant27/1 -> Mult27/1
  Mult24/1 -> AddSub21/2
  Constant28/1 -> Mult28/1
  Delay27/1 -> Mult31/2
  Constant31/1 -> Mult31/1
  Constant24/1 -> Mult24/1
  Constant30/1 -> Mult30/1
  Constant26/1 -> Mult26/1
  Mult31/1 -> AddSub27/1
  AddSub26/1 -> AddSub27/2
  AddSub27/1 -> Out4/1

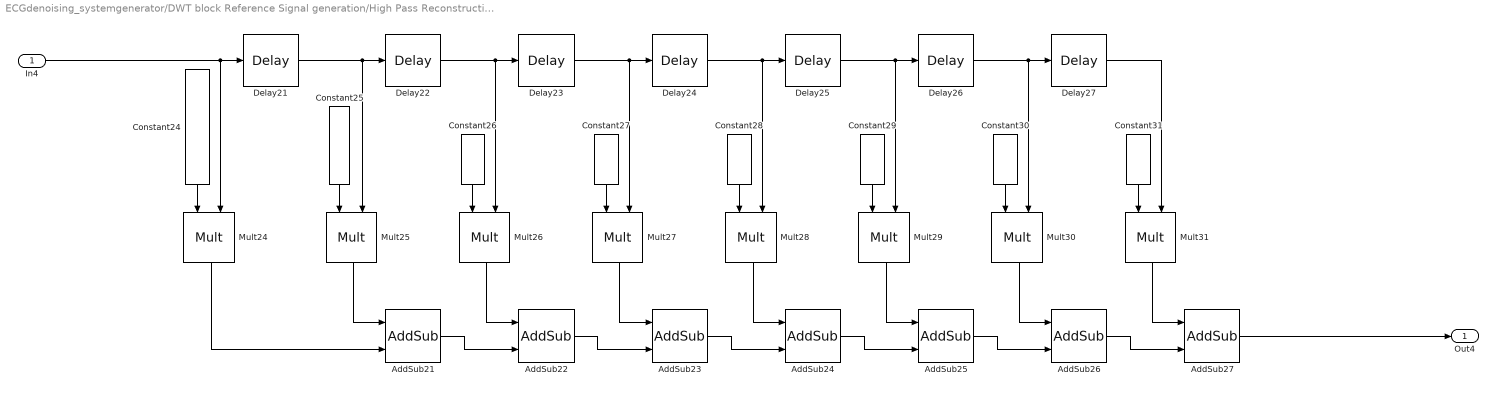
== system ECGdenoising_systemgenerator/DWT block Reference Signal generation/High Pass Reconstruction5 ==
  In4 : Inport
  AddSub{21..27} (7 alike) : xbsIndex_r4/AddSub  mode=Addition  use_carryin=off  use_carryout=off  en=off  latency=0  precision=User Defined  arith_type="Signed  (2's comp)"  n_bits=16  bin_pt=14  quantization=Truncate  overflow=Saturate  use_behavioral_HDL=off  hw_selection=Fabric  pipelined=off  dbl_ovrd=off  block_type=addsub
  Constant24 : xbsIndex_r4/Constant  const=-0.0105974018  gui_display_data_type=Fixed-point  arith_type=Signed (2's comp)  n_bits=16  bin_pt=14  preci_type=Single  exp_width=8  frac_width=24  explicit_period=on  period=2  equ=P=C  opselect=C  inp2=PCIN>>17  opr=+  inp1=P  carry=CIN  dbl_ovrd=off  block_type=constant
  Constant25 : xbsIndex_r4/Constant  const=-0.032883011  gui_display_data_type=Fixed-point  arith_type=Signed (2's comp)  n_bits=16  bin_pt=14  preci_type=Single  exp_width=8  frac_width=24  explicit_period=on  period=2  equ=P=C  opselect=C  inp2=PCIN>>17  opr=+  inp1=P  carry=CIN  dbl_ovrd=off  block_type=constant
  Constant26 : xbsIndex_r4/Constant  const=0.0308413818  gui_display_data_type=Fixed-point  arith_type=Signed (2's comp)  n_bits=16  bin_pt=14  preci_type=Single  exp_width=8  frac_width=24  explicit_period=on  period=2  equ=P=C  opselect=C  inp2=PCIN>>17  opr=+  inp1=P  carry=CIN  dbl_ovrd=off  block_type=constant
  Constant27 : xbsIndex_r4/Constant  const=0.1870348117  gui_display_data_type=Fixed-point  arith_type=Signed (2's comp)  n_bits=16  bin_pt=14  preci_type=Single  exp_width=8  frac_width=24  explicit_period=on  period=2  equ=P=C  opselect=C  inp2=PCIN>>17  opr=+  inp1=P  carry=CIN  dbl_ovrd=off  block_type=constant
  Constant28 : xbsIndex_r4/Constant  const=-0.0279837694  gui_display_data_type=Fixed-point  arith_type=Signed (2's comp)  n_bits=16  bin_pt=14  preci_type=Single  exp_width=8  frac_width=24  explicit_period=on  period=2  equ=P=C  opselect=C  inp2=PCIN>>17  opr=+  inp1=P  carry=CIN  dbl_ovrd=off  block_type=constant
  Constant29 : xbsIndex_r4/Constant  const=-0.6308807679  gui_display_data_type=Fixed-point  arith_type=Signed (2's comp)  n_bits=16  bin_pt=14  preci_type=Single  exp_width=8  frac_width=24  explicit_period=on  period=2  equ=P=C  opselect=C  inp2=PCIN>>17  opr=+  inp1=P  carry=CIN  dbl_ovrd=off  block_type=constant
  Constant30 : xbsIndex_r4/Constant  const=0.7148465706  gui_display_data_type=Fixed-point  arith_type=Signed (2's comp)  n_bits=16  bin_pt=14  preci_type=Single  exp_width=8  frac_width=24  explicit_period=on  period=2  equ=P=C  opselect=C  inp2=PCIN>>17  opr=+  inp1=P  carry=CIN  dbl_ovrd=off  block_type=constant
  Constant31 : xbsIndex_r4/Constant  const=-0.2303778133  gui_display_data_type=Fixed-point  arith_type=Signed (2's comp)  n_bits=16  bin_pt=14  preci_type=Single  exp_width=8  frac_width=24  explicit_period=on  period=2  equ=P=C  opselect=C  inp2=PCIN>>17  opr=+  inp1=P  carry=CIN  dbl_ovrd=off  block_type=constant
  Delay{21..27} (7 alike) : xbsIndex_r4/Delay  rst=off  infoeditControl=Selection of Reset will increase slice count due to use of real FFs and instead of SRLs  en=off  latency=1  reg_retiming=off  dbl_ovrd=off  block_type=delay
      settings: infoedit=Hardware notes: A delay line is a chain, each link of which is an SRL16 or SRL32 followed by a flip-flop.
  Mult{24..31} (8 alike) : xbsIndex_r4/Mult  precision=User Defined  arith_type="Signed  (2's comp)"  n_bits=32  bin_pt=28  quantization=Truncate  overflow=Saturate  en=off  latency=0  use_behavioral_HDL=off  opt=Speed  use_embedded=on  optimum_pipeline=off  pipeline=on  dbl_ovrd=off  use_rpm=on  placement_style=Triangular  block_type=mult
  Out4 : Outport
  wires:
  Delay21/1 -> Mult25/2, Delay22/1
  Delay22/1 -> Mult26/2, Delay23/1
  Delay23/1 -> Mult27/2, Delay24/1
  AddSub21/1 -> AddSub22/2
  AddSub23/1 -> AddSub24/2
  In4/1 -> Mult24/2, Delay21/1
  Mult29/1 -> AddSub25/1
  Constant25/1 -> Mult25/1
  Delay24/1 -> Mult28/2, Delay25/1
  Mult27/1 -> AddSub23/1
  Mult28/1 -> AddSub24/1
  AddSub24/1 -> AddSub25/2
  Mult26/1 -> AddSub22/1
  Delay26/1 -> Mult30/2, Delay27/1
  AddSub22/1 -> AddSub23/2
  Delay25/1 -> Mult29/2, Delay26/1
  Mult25/1 -> AddSub21/1
  Mult30/1 -> AddSub26/1
  AddSub25/1 -> AddSub26/2
  Constant29/1 -> Mult29/1
  Constant27/1 -> Mult27/1
  Mult24/1 -> AddSub21/2
  Constant28/1 -> Mult28/1
  Delay27/1 -> Mult31/2
  Constant31/1 -> Mult31/1
  Constant24/1 -> Mult24/1
  Constant30/1 -> Mult30/1
  Constant26/1 -> Mult26/1
  Mult31/1 -> AddSub27/1
  AddSub26/1 -> AddSub27/2
  AddSub27/1 -> Out4/1

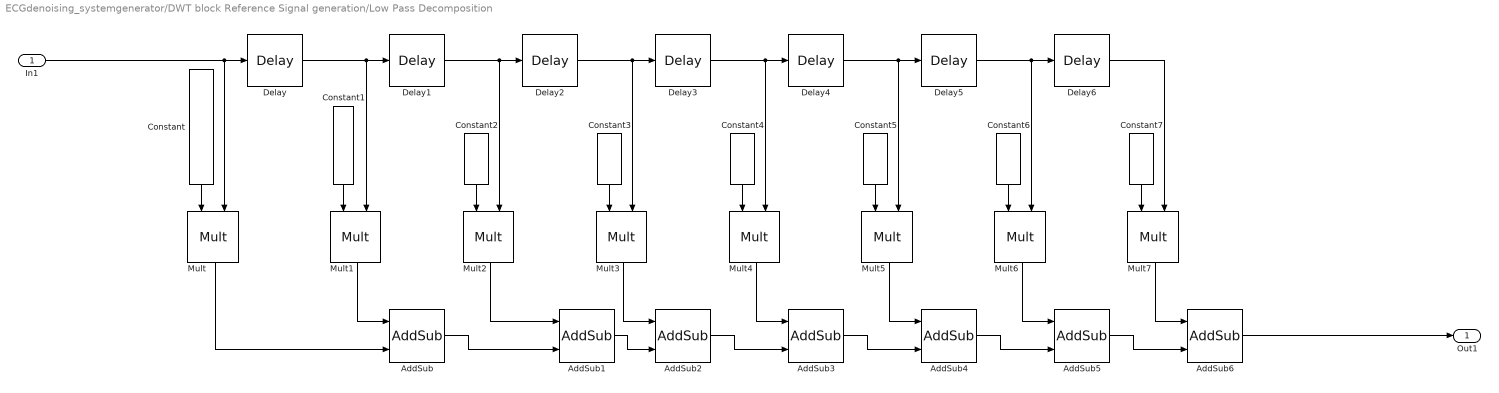
== system ECGdenoising_systemgenerator/DWT block Reference Signal generation/Low Pass Decomposition  ==
  In1 : Inport
  AddSub{,1..6} (7 alike) : xbsIndex_r4/AddSub  mode=Addition  use_carryin=off  use_carryout=off  en=off  latency=0  precision=User Defined  arith_type="Signed  (2's comp)"  n_bits=16  bin_pt=14  quantization=Truncate  overflow=Saturate  use_behavioral_HDL=off  hw_selection=Fabric  pipelined=off  dbl_ovrd=off  block_type=addsub
  Constant : xbsIndex_r4/Constant  const=-0.0105974018  gui_display_data_type=Fixed-point  arith_type=Signed (2's comp)  n_bits=16  bin_pt=14  preci_type=Single  exp_width=8  frac_width=24  explicit_period=on  period=1  equ=P=C  opselect=C  inp2=PCIN>>17  opr=+  inp1=P  carry=CIN  dbl_ovrd=off  block_type=constant
  Constant1 : xbsIndex_r4/Constant  const=0.0328830117  gui_display_data_type=Fixed-point  arith_type=Signed (2's comp)  n_bits=16  bin_pt=14  preci_type=Single  exp_width=8  frac_width=24  explicit_period=on  period=1  equ=P=C  opselect=C  inp2=PCIN>>17  opr=+  inp1=P  carry=CIN  dbl_ovrd=off  block_type=constant
  Constant2 : xbsIndex_r4/Constant  const=0.0308413818  gui_display_data_type=Fixed-point  arith_type=Signed (2's comp)  n_bits=16  bin_pt=14  preci_type=Single  exp_width=8  frac_width=24  explicit_period=on  period=1  equ=P=C  opselect=C  inp2=PCIN>>17  opr=+  inp1=P  carry=CIN  dbl_ovrd=off  block_type=constant
  Constant3 : xbsIndex_r4/Constant  const=-0.1870348117  gui_display_data_type=Fixed-point  arith_type=Signed (2's comp)  n_bits=16  bin_pt=14  preci_type=Single  exp_width=8  frac_width=24  explicit_period=on  period=1  equ=P=C  opselect=C  inp2=PCIN>>17  opr=+  inp1=P  carry=CIN  dbl_ovrd=off  block_type=constant
  Constant4 : xbsIndex_r4/Constant  const=-0.0279837694  gui_display_data_type=Fixed-point  arith_type=Signed (2's comp)  n_bits=16  bin_pt=14  preci_type=Single  exp_width=8  frac_width=24  explicit_period=on  period=1  equ=P=C  opselect=C  inp2=PCIN>>17  opr=+  inp1=P  carry=CIN  dbl_ovrd=off  block_type=constant
  Constant5 : xbsIndex_r4/Constant  const=0.6308807679  gui_display_data_type=Fixed-point  arith_type=Signed (2's comp)  n_bits=16  bin_pt=14  preci_type=Single  exp_width=8  frac_width=24  explicit_period=on  period=1  equ=P=C  opselect=C  inp2=PCIN>>17  opr=+  inp1=P  carry=CIN  dbl_ovrd=off  block_type=constant
  Constant6 : xbsIndex_r4/Constant  const=0.7148465706  gui_display_data_type=Fixed-point  arith_type=Signed (2's comp)  n_bits=16  bin_pt=14  preci_type=Single  exp_width=8  frac_width=24  explicit_period=on  period=1  equ=P=C  opselect=C  inp2=PCIN>>17  opr=+  inp1=P  carry=CIN  dbl_ovrd=off  block_type=constant
  Constant7 : xbsIndex_r4/Constant  const=0.2303778133  gui_display_data_type=Fixed-point  arith_type=Signed (2's comp)  n_bits=16  bin_pt=14  preci_type=Single  exp_width=8  frac_width=24  explicit_period=on  period=1  equ=P=C  opselect=C  inp2=PCIN>>17  opr=+  inp1=P  carry=CIN  dbl_ovrd=off  block_type=constant
  Delay{,1..6} (7 alike) : xbsIndex_r4/Delay  rst=off  infoeditControl=Selection of Reset will increase slice count due to use of real FFs and instead of SRLs  en=off  latency=1  reg_retiming=off  dbl_ovrd=off  block_type=delay
      settings: infoedit=Hardware notes: A delay line is a chain, each link of which is an SRL16 or SRL32 followed by a flip-flop.
  Mult{,1..7} (8 alike) : xbsIndex_r4/Mult  precision=User Defined  arith_type="Signed  (2's comp)"  n_bits=32  bin_pt=28  quantization=Truncate  overflow=Saturate  en=off  latency=0  use_behavioral_HDL=off  opt=Speed  use_embedded=on  optimum_pipeline=off  pipeline=on  dbl_ovrd=off  use_rpm=on  placement_style=Triangular  block_type=mult
  Out1 : Outport
  wires:
  AddSub6/1 -> Out1/1
  Constant7/1 -> Mult7/1
  Mult6/1 -> AddSub5/1
  AddSub4/1 -> AddSub5/2
  AddSub5/1 -> AddSub6/2
  Constant6/1 -> Mult6/1
  Delay6/1 -> Mult7/2
  Delay5/1 -> Mult6/2, Delay6/1
  AddSub3/1 -> AddSub4/2
  Mult7/1 -> AddSub6/1
  Constant/1 -> Mult/1
  Delay/1 -> Mult1/2, Delay1/1
  AddSub/1 -> AddSub1/2
  Constant3/1 -> Mult3/1
  AddSub1/1 -> AddSub2/2
  Delay3/1 -> Mult4/2, Delay4/1
  Constant4/1 -> Mult4/1
  Mult4/1 -> AddSub3/1
  Delay4/1 -> Mult5/2, Delay5/1
  Constant5/1 -> Mult5/1
  Constant2/1 -> Mult2/1
  AddSub2/1 -> AddSub3/2
  Mult5/1 -> AddSub4/1
  Constant1/1 -> Mult1/1
  Mult/1 -> AddSub/2
  Delay1/1 -> Mult2/2, Delay2/1
  Mult2/1 -> AddSub1/1
  Delay2/1 -> Mult3/2, Delay3/1
  Mult1/1 -> AddSub/1
  Mult3/1 -> AddSub2/1
  In1/1 -> Mult/2, Delay/1

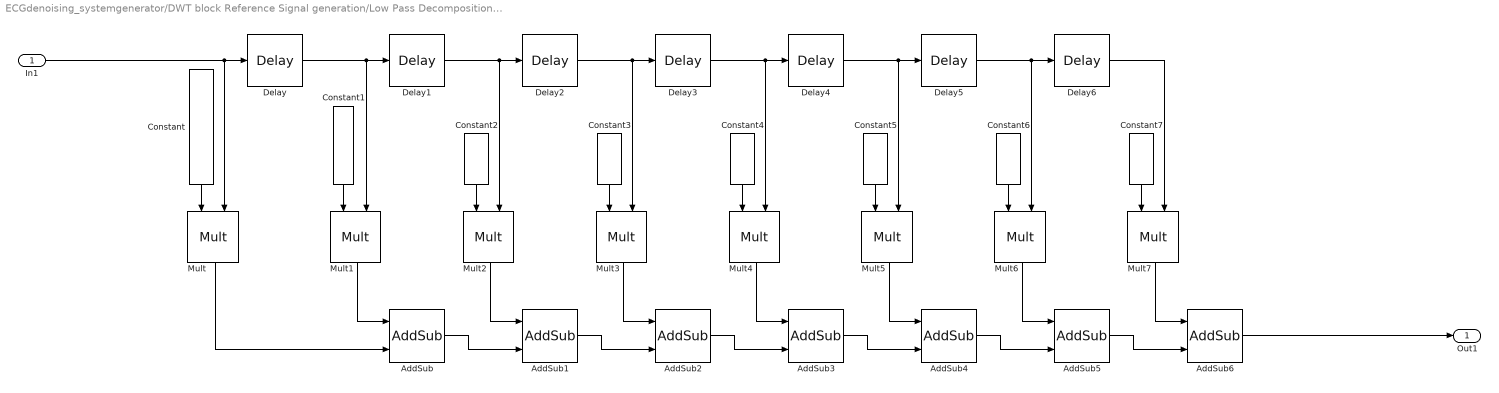
== system ECGdenoising_systemgenerator/DWT block Reference Signal generation/Low Pass Decomposition 1 ==
  In1 : Inport
  AddSub{,1..6} (7 alike) : xbsIndex_r4/AddSub  mode=Addition  use_carryin=off  use_carryout=off  en=off  latency=0  precision=User Defined  arith_type="Signed  (2's comp)"  n_bits=16  bin_pt=14  quantization=Truncate  overflow=Saturate  use_behavioral_HDL=off  hw_selection=Fabric  pipelined=off  dbl_ovrd=off  block_type=addsub
  Constant : xbsIndex_r4/Constant  const=-0.0105974018  gui_display_data_type=Fixed-point  arith_type=Signed (2's comp)  n_bits=16  bin_pt=14  preci_type=Single  exp_width=8  frac_width=24  explicit_period=on  period=2  equ=P=C  opselect=C  inp2=PCIN>>17  opr=+  inp1=P  carry=CIN  dbl_ovrd=off  block_type=constant
  Constant1 : xbsIndex_r4/Constant  const=0.0328830117  gui_display_data_type=Fixed-point  arith_type=Signed (2's comp)  n_bits=16  bin_pt=14  preci_type=Single  exp_width=8  frac_width=24  explicit_period=on  period=2  equ=P=C  opselect=C  inp2=PCIN>>17  opr=+  inp1=P  carry=CIN  dbl_ovrd=off  block_type=constant
  Constant2 : xbsIndex_r4/Constant  const=0.0308413818  gui_display_data_type=Fixed-point  arith_type=Signed (2's comp)  n_bits=16  bin_pt=14  preci_type=Single  exp_width=8  frac_width=24  explicit_period=on  period=2  equ=P=C  opselect=C  inp2=PCIN>>17  opr=+  inp1=P  carry=CIN  dbl_ovrd=off  block_type=constant
  Constant3 : xbsIndex_r4/Constant  const=-0.1870348117  gui_display_data_type=Fixed-point  arith_type=Signed (2's comp)  n_bits=16  bin_pt=14  preci_type=Single  exp_width=8  frac_width=24  explicit_period=on  period=2  equ=P=C  opselect=C  inp2=PCIN>>17  opr=+  inp1=P  carry=CIN  dbl_ovrd=off  block_type=constant
  Constant4 : xbsIndex_r4/Constant  const=-0.0279837694  gui_display_data_type=Fixed-point  arith_type=Signed (2's comp)  n_bits=16  bin_pt=14  preci_type=Single  exp_width=8  frac_width=24  explicit_period=on  period=2  equ=P=C  opselect=C  inp2=PCIN>>17  opr=+  inp1=P  carry=CIN  dbl_ovrd=off  block_type=constant
  Constant5 : xbsIndex_r4/Constant  const=0.6308807679  gui_display_data_type=Fixed-point  arith_type=Signed (2's comp)  n_bits=16  bin_pt=14  preci_type=Single  exp_width=8  frac_width=24  explicit_period=on  period=2  equ=P=C  opselect=C  inp2=PCIN>>17  opr=+  inp1=P  carry=CIN  dbl_ovrd=off  block_type=constant
  Constant6 : xbsIndex_r4/Constant  const=0.7148465706  gui_display_data_type=Fixed-point  arith_type=Signed (2's comp)  n_bits=16  bin_pt=14  preci_type=Single  exp_width=8  frac_width=24  explicit_period=on  period=2  equ=P=C  opselect=C  inp2=PCIN>>17  opr=+  inp1=P  carry=CIN  dbl_ovrd=off  block_type=constant
  Constant7 : xbsIndex_r4/Constant  const=0.2303778133  gui_display_data_type=Fixed-point  arith_type=Signed (2's comp)  n_bits=16  bin_pt=14  preci_type=Single  exp_width=8  frac_width=24  explicit_period=on  period=2  equ=P=C  opselect=C  inp2=PCIN>>17  opr=+  inp1=P  carry=CIN  dbl_ovrd=off  block_type=constant
  Delay{,1..6} (7 alike) : xbsIndex_r4/Delay  rst=off  infoeditControl=Selection of Reset will increase slice count due to use of real FFs and instead of SRLs  en=off  latency=1  reg_retiming=off  dbl_ovrd=off  block_type=delay
      settings: infoedit=Hardware notes: A delay line is a chain, each link of which is an SRL16 or SRL32 followed by a flip-flop.
  Mult{,1..7} (8 alike) : xbsIndex_r4/Mult  precision=User Defined  arith_type="Signed  (2's comp)"  n_bits=32  bin_pt=28  quantization=Truncate  overflow=Saturate  en=off  latency=0  use_behavioral_HDL=off  opt=Speed  use_embedded=on  optimum_pipeline=off  pipeline=on  dbl_ovrd=off  use_rpm=on  placement_style=Triangular  block_type=mult
  Out1 : Outport
  wires:
  AddSub6/1 -> Out1/1
  Constant7/1 -> Mult7/1
  Mult6/1 -> AddSub5/1
  AddSub4/1 -> AddSub5/2
  AddSub5/1 -> AddSub6/2
  Constant6/1 -> Mult6/1
  Delay6/1 -> Mult7/2
  Delay5/1 -> Mult6/2, Delay6/1
  AddSub3/1 -> AddSub4/2
  Mult7/1 -> AddSub6/1
  Constant/1 -> Mult/1
  Delay/1 -> Mult1/2, Delay1/1
  AddSub/1 -> AddSub1/2
  Constant3/1 -> Mult3/1
  AddSub1/1 -> AddSub2/2
  Delay3/1 -> Mult4/2, Delay4/1
  Constant4/1 -> Mult4/1
  Mult4/1 -> AddSub3/1
  Delay4/1 -> Mult5/2, Delay5/1
  Constant5/1 -> Mult5/1
  Constant2/1 -> Mult2/1
  AddSub2/1 -> AddSub3/2
  Mult5/1 -> AddSub4/1
  Constant1/1 -> Mult1/1
  Mult/1 -> AddSub/2
  Delay1/1 -> Mult2/2, Delay2/1
  Mult2/1 -> AddSub1/1
  Delay2/1 -> Mult3/2, Delay3/1
  Mult1/1 -> AddSub/1
  Mult3/1 -> AddSub2/1
  In1/1 -> Mult/2, Delay/1
